simulink model "hexAddFmTestHarness"  (R2024a)
settings: configuration reference "standardSILConfiguraitonParams" (kept outside this file)
settings Model: Creator=jerem  LastModifiedBy=jerem
settings ConfigSetRef: SourceName=standardSILConfiguraitonParams  SourceLocation=Base Workspace

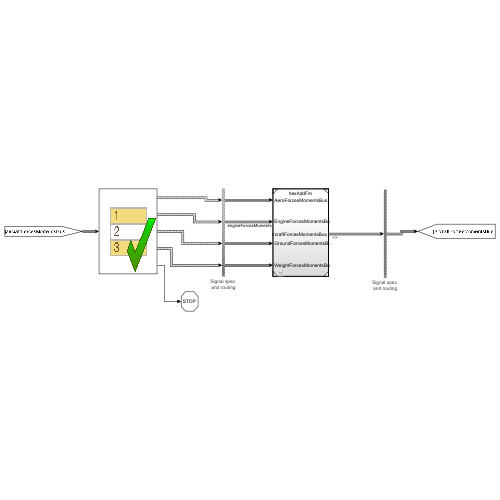
[thumbnail: Simulink's stored preview of the top-level diagram]
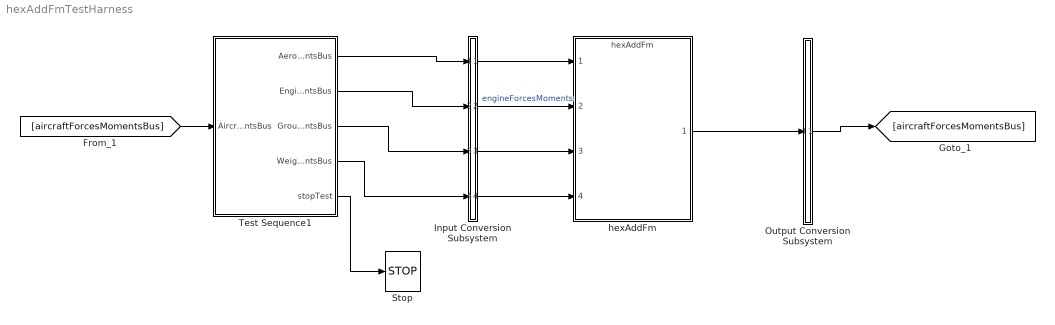
== system hexAddFmTestHarness ==
  Input Conversion Subsystem : Subsystem  Tag=__SLT_ICS__  Description=|
      | Signal spec.
      | and routing
      settings: AttributesFormatString=%<Description>
  Output Conversion Subsystem : Subsystem  Tag=__SLT_OCS__  Description=|
      | Signal spec.
      | and routing
      mask init:
      | ICDictionary = get_param(bdroot, 'DataDictionary');
      | if isempty(ICDictionary)
      |    ICScope = Simulink.data.BaseWorkspace;
      | else
      |    ICScope = Simulink.data.DataDictionary(ICDictionary);
      | end
      | 
      | IC1 = Simulink.Bus.createMATLABStruct('AircraftForcesMomentsBus', [], [1 1], ICScope);
      settings: AttributesFormatString=%<Description>
  Stop : Stop
  Test Sequence1 : Test Sequence  TreatAsAtomicUnit=on
  hexAddFm : ModelReference  ModelNameDialog=hexAddFm  SimulationMode=Normal  ModelReferenceVersion=1.14
  wires:
  Test Sequence1/1(AeroForcesMomentsBus) -> Input Conversion Subsystem/1(Inport_1)
  Test Sequence1/2(EngineForcesMomentsBus) -> Input Conversion Subsystem/2(Inport_2)
  Test Sequence1/3(GroundForcesMomentsBus) -> Input Conversion Subsystem/3(Inport_3)
  Test Sequence1/4(WeightForcesMomentsBus) -> Input Conversion Subsystem/4(Inport_4)
  [aircraftForcesMomentsBus] -> Test Sequence1/1(AircraftForcesMomentsBus)
  Output Conversion Subsystem/1(Outport_1) -> [aircraftForcesMomentsBus]
  Test Sequence1/5(stopTest) -> Stop/1
  hexAddFm/1 -> Output Conversion Subsystem/1(Inport_1)
  Input Conversion Subsystem/1(Outport_1) -> hexAddFm/1
  Input Conversion Subsystem/2(Outport_2) -> hexAddFm/2  "engineForcesMoments"
  Input Conversion Subsystem/3(Outport_3) -> hexAddFm/3
  Input Conversion Subsystem/4(Outport_4) -> hexAddFm/4

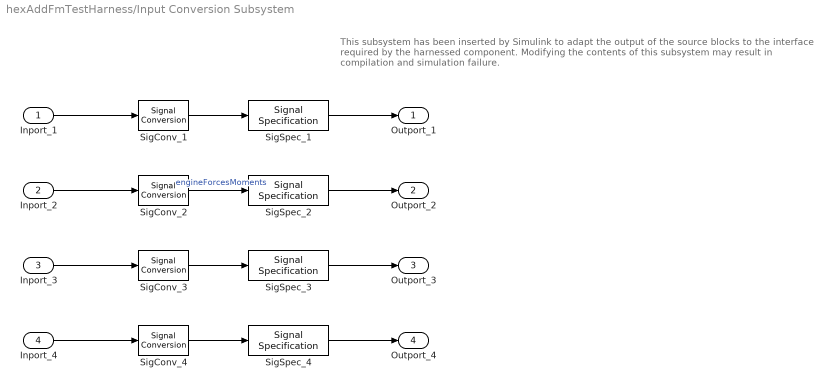
== system hexAddFmTestHarness/Input Conversion Subsystem ==
  note: This subsystem has been inserted by Simulink to adapt the output of the source blocks to the interface required by the harnessed component.
      |  Modifying the contents of this subsystem may result in compilation and simulation failure.
  Inport_1 : Inport
  Inport_2 : Inport  Port=2
  Inport_3 : Inport  Port=3
  Inport_4 : Inport  Port=4
  SigConv_{1..4} (4 alike) : SignalConversion  ConversionOutput=Virtual bus  OverrideOpt=off
  SigSpec_{1..4} (4 alike) : SignalSpecification  OutDataTypeStr=Bus: ComponentForcesMomentsBus
  Outport_1 : Outport
  Outport_2 : Outport  Port=2
  Outport_3 : Outport  Port=3
  Outport_4 : Outport  Port=4
  wires:
  SigSpec_1/1 -> Outport_1/1
  SigConv_1/1 -> SigSpec_1/1
  Inport_1/1 -> SigConv_1/1
  SigSpec_2/1 -> Outport_2/1
  SigConv_2/1 -> SigSpec_2/1  "engineForcesMoments"
  Inport_2/1 -> SigConv_2/1
  SigSpec_3/1 -> Outport_3/1
  SigConv_3/1 -> SigSpec_3/1
  Inport_3/1 -> SigConv_3/1
  SigSpec_4/1 -> Outport_4/1
  SigConv_4/1 -> SigSpec_4/1
  Inport_4/1 -> SigConv_4/1

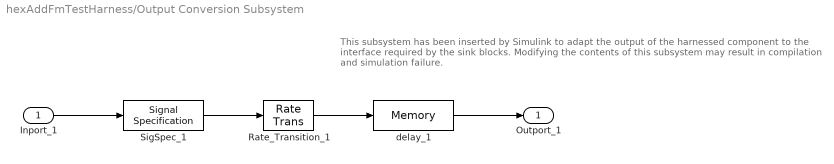
== system hexAddFmTestHarness/Output Conversion Subsystem ==
  note: This subsystem has been inserted by Simulink to adapt the output of the harnessed component to the interface required by the sink blocks.
      |  Modifying the contents of this subsystem may result in compilation and simulation failure.
  Inport_1 : Inport
  Rate_Transition_1 : RateTransition  OutPortSampleTimeOpt=Inherit
  SigSpec_1 : SignalSpecification  OutDataTypeStr=Bus: AircraftForcesMomentsBus  Dimensions=[1]
  delay_1 : Memory  InitialCondition=IC1
  Outport_1 : Outport
  wires:
  Inport_1/1 -> SigSpec_1/1
  SigSpec_1/1 -> Rate_Transition_1/1
  Rate_Transition_1/1 -> delay_1/1
  delay_1/1 -> Outport_1/1

== stateflow chart hexAddFmTestHarness/Test Sequence1 ==
  state Scenario_1
    state Initialize
      %% Initialize data outputs.
      stopTest = false;
      AeroForcesMomentsBus.forcesInBody_N = zeros(3,1);
      AeroForcesMomentsBus.momentsInBody_Nm = zeros(3,1);
      EngineForcesMomentsBus.forcesInBody_N = zeros(3,1);
      EngineForcesMomentsBus.momentsInBody_Nm = zeros(3,1);
      GroundForcesMomentsBus.forcesInBody_N = zeros(3,1);
      GroundForcesMomentsBus.momentsInBody_Nm = zeros(3,1);
      WeightForcesMomentsBus.forcesInBody_N = zeros(3,1);
      WeightForcesMomentsBus.momentsInBody_Nm = zeros(3,1);
      randomInputs = rand(48,1);
    state Define_Test1_Inputs
      % set to random values
      AeroForcesMomentsBus.forcesInBody_N = randomInputs(1:3);
      AeroForcesMomentsBus.momentsInBody_Nm = randomInputs(4:6);
      EngineForcesMomentsBus.forcesInBody_N = randomInputs(7:9);
      EngineForcesMomentsBus.momentsInBody_Nm = randomInputs(10:12);
      GroundForcesMomentsBus.forcesInBody_N = randomInputs(13:15);
      GroundForcesMomentsBus.momentsInBody_Nm = randomInputs(16:18);
      WeightForcesMomentsBus.forcesInBody_N = randomInputs(19:21);
      WeightForcesMomentsBus.momentsInBody_Nm = randomInputs(22:24);
    state Test1
      % Test 1: Check AircraftForcesMomentsBus is the sum of AeroForcesMomentsBus, EngineForcesMomentsBus, and GroundForcesMomentsBus
      verify(all(isClose(AircraftForcesMomentsBus.forcesInBody_N, AeroForcesMomentsBus.forcesInBody_N + EngineForcesMomentsBus.forcesInBody_N + GroundForcesMomentsBus.forcesInBody_N + WeightForcesMomentsBus.forcesInBody_N)))
      verify(all(isClose(AircraftForcesMomentsBus.momentsInBody_Nm, EngineForcesMomentsBus.momentsInBody_Nm + AeroForcesMomentsBus.momentsInBody_Nm + WeightForcesMomentsBus.momentsInBody_Nm + GroundForcesMomentsBus.momentsInBody_Nm)))
    state Define_Test2_Inputs
      % set to random values
      AeroForcesMomentsBus.forcesInBody_N = randomInputs(25:27);
      AeroForcesMomentsBus.momentsInBody_Nm = randomInputs(28:30);
      EngineForcesMomentsBus.forcesInBody_N = randomInputs(31:33);
      EngineForcesMomentsBus.momentsInBody_Nm = randomInputs(34:36);
      GroundForcesMomentsBus.forcesInBody_N = randomInputs(37:39);
      GroundForcesMomentsBus.momentsInBody_Nm = randomInputs(40:42);
      WeightForcesMomentsBus.forcesInBody_N = randomInputs(43:45);
      WeightForcesMomentsBus.momentsInBody_Nm = randomInputs(46:48);
    state Test2
      % Test 2: Same as test 1 but with another set of random inputs
      verify(all(isClose(AircraftForcesMomentsBus.forcesInBody_N, AeroForcesMomentsBus.forcesInBody_N + EngineForcesMomentsBus.forcesInBody_N + GroundForcesMomentsBus.forcesInBody_N + WeightForcesMomentsBus.forcesInBody_N)))
      verify(all(isClose(AircraftForcesMomentsBus.momentsInBody_Nm, AeroForcesMomentsBus.momentsInBody_Nm + EngineForcesMomentsBus.momentsInBody_Nm + WeightForcesMomentsBus.momentsInBody_Nm + GroundForcesMomentsBus.momentsInBody_Nm)))
    state EndTest
      stopTest = true;
    (default) -> Initialize
    Initialize -> Define_Test1_Inputs : [
        | true
        | ]
    Define_Test1_Inputs -> Test1 : [
        | after(1,sec)
        | ]
    Test1 -> Define_Test2_Inputs : [
        | true
        | ]
    Define_Test2_Inputs -> Test2 : [
        | after(1,sec)
        | ]
    Test2 -> EndTest : [
        | true
        | ]
  (default) -> Scenario_1 : {assert(Active_Scenario_Index == 1,'The value of Scenario Parameter ''Active_Scenario_Index'' is not valid. Use the index of the scenario to specify it.')}
  data: AircraftForcesMomentsBus input Bus: AircraftForcesMomentsBus size=[1]; AeroForcesMomentsBus output Bus: ComponentForcesMomentsBus size=[1]; EngineForcesMomentsBus output Bus: ComponentForcesMomentsBus size=[1]; GroundForcesMomentsBus output Bus: ComponentForcesMomentsBus size=[1]; Active_Scenario_Index parameter =1; randomInputs local; WeightForcesMomentsBus output Bus: ComponentForcesMomentsBus size=[1]; stopTest output
